simulink model "psbtransfosat"  (Simulink 6.0)
settings: Solver=ode15s  SolverMode=SingleTasking  StartTime=0.0  StopTime=0.5  RelTol=1e-3  AbsTol=1e-2
InitFcn:
  | powericon('psbinitsys',bdroot);
undefined symbols (not defined in the file or in its folder): D1, Delta
libraries: powerlib2 x10, powerlib_extras x1
settings Model: Creator=patrice  LastModifiedBy=batserve  ExtModeTrigMode=oneshot  ExtModeArmWhenConnect=off  ExtModeAutoUpdateStatusClock=off
settings DataIOCC: LimitDataPoints=off  SignalLoggingName=sigsOut
settings OptimizationCC: BlockReduction=off  BooleanDataType=off
settings DebuggingCC: CheckExecutionContextPreStartOutputMsg=on  CheckExecutionContextRuntimeOutputMsg=on  SolverPrmCheckMsg=none  IntegerOverflowMsg=none
settings HardwareCC: TargetUnknown=on
settings RTWCC: TemplateMakefile=grt_unix.tmf

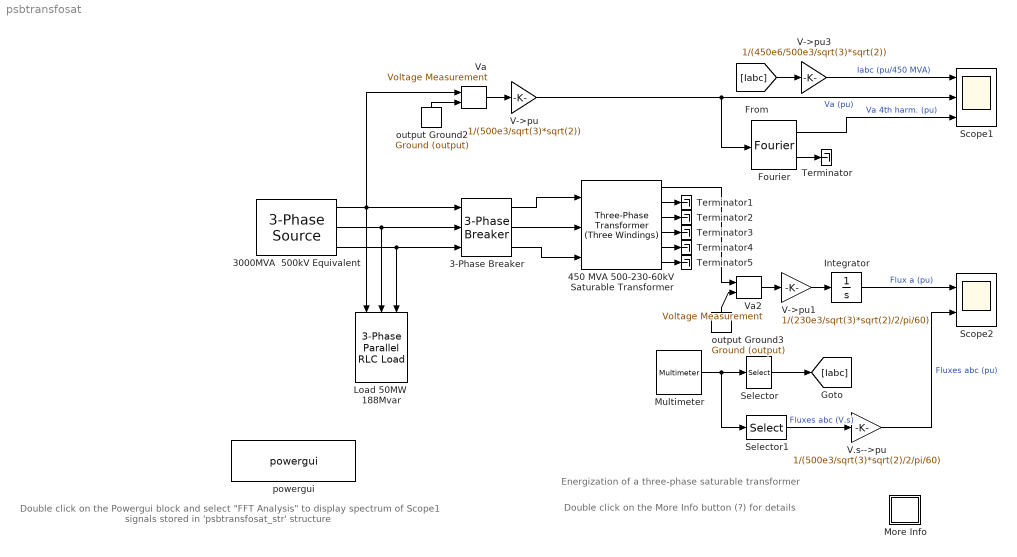
== system psbtransfosat ==
  note: Energization of a three-phase saturable transformer
  note: Double click on the More Info button (?) for details
  note: Double click on the Powergui block and select
      |  "FFT Analysis" to display spectrum of Scope1 signals
      |  stored in 'psbtransfosat_str' structure
  3-Phase Breaker : powerlib2/Elements/3-Phase Breaker  init_states=open  sa=on  sb=on  sc=on  sw_times=[0.05]  Ts=0  comext=off  Ron=0.01  Rp=100e6  Cp=inf  mesure=Breaker currents
  3000MVA  500kV Equivalent : powerlib2/Electrical Sources/3-Phase Source  Tag=PoWeRsYsTeMbLoCk  V=500e3  Phi=0  F=60  InternalConnection=Yg  RLoff=off  R=5.55  L=0.221  Psc=0  Vbase=0  XRratio=0  PSBOutputType=111
  450 MVA 500-230-60kV Saturable Transformer : powerlib2/Elements/Three-Phase Transformer (Three Windings)  Tag=PoWeRsYsTeMbLoCk  confi=ABC as input terminals  nom=[ 450e6 , 60 ]  ydw1=Yg  w1=[ 500e3 0.002 0.08 ]  ydw2=Yg  w2=[ 230e3 0.002 0.08]  ydw3=Delta (D1)  w3=[ 60e3 0.015 0.30]  ynsat=on  rmag=500  lm=500  sat="[0 0; 0.0 1.2; 1.0  1.52]"  hyst=off  matfile='hysteresis'  sif=on  ifl=[0.8 -0.4 0.4]  initialslopes=[+1 +1 +1]  mesure=Fluxes and magnetization currents ( Imag )  PSBOutputType=1111111
  Fourier : powerlib_extras/Measurements/Fourier  f1=60  n=4
  Integrator : Integrator  InitialCondition=0.8  ZeroCross=off
  Load 50MW  188Mvar : powerlib2/Elements/3-Phase Parallel RLC Load  Orientation=down  Vpp=500e3  fn=60  P3=50e6  QL3=0  QC3=188e6
  More Info : Subsystem
      mask Display: disp('?')
  Multimeter : powerlib2/Measurements/Multimeter  Tag=PoWeRsYsTeMmEaSuReMeNt  PhasorSimulation=off  OutputType=Magnitude  sel=[1 2 3 7 8 9]  L=9  Gain=[1 1 1 1 1 1]  yselected={'Ib: 3-Phase Breaker/Breaker A','Ib: 3-Phase Breaker/Breaker B','Ib: 3-Phase Breaker/Breaker C','Flux_A: 450 MVA 500-230-60kV Saturable Transformer','Flux_B: 450 MVA 500-230-60kV Saturable Transformer','Flux_C: 450 MVA 500-230-60kV Saturable Transformer'};  PSBOutputType=1  PSBequivalent=0  AxesSetting=[0,0.1,-100,100]  Display=0  SavedBlockNames={}
  Scope1 : Scope  NumInputPorts=3
      settings: TimeRange=0.5  YMin=-1.5~-1.5~0.05  YMax=3~1.25~0.25  SaveName=psbtransfosat_str  SampleInput=on  SampleTime=1/60/333
  Scope2 : Scope  NumInputPorts=2
      settings: TimeRange=0.5  YMin=-1~-2  YMax=3~3  DataFormat=Structure
  Selector : Selector  Elements=1:3  InputPortWidth=6
  Selector1 : Selector  Elements=4:6  InputPortWidth=6
  Terminator{,1..5} (6 alike) : Terminator
  V->pu : Gain  Gain=1/(500e3/sqrt(3)*sqrt(2))  SaturateOnIntegerOverflow=on
  V->pu1 : Gain  Gain=1/(230e3/sqrt(3)*sqrt(2)/2/pi/60)  SaturateOnIntegerOverflow=on
  V->pu3 : Gain  Gain=1/(450e6/500e3/sqrt(3)*sqrt(2))  SaturateOnIntegerOverflow=on
  V.s-->pu : Gain  Gain=1/(500e3/sqrt(3)*sqrt(2)/2/pi/60)  SaturateOnIntegerOverflow=on
  Va : powerlib2/Measurements/Voltage Measurement  Tag=PoWeRsYsTeMmEaSuReMeNt  PhasorSimulation=off  OutputType=Magnitude  PSBOutputType=0  PSBequivalent=0
  Va2 : powerlib2/Measurements/Voltage Measurement  Tag=PoWeRsYsTeMmEaSuReMeNt  PhasorSimulation=off  OutputType=Magnitude  PSBOutputType=0  PSBequivalent=1
  output Ground2 : powerlib2/Connectors/Ground (output)  Tag=PoWeRsYsTeMbLoCk  Orientation=up  PSBOutputType=1
  output Ground3 : powerlib2/Connectors/Ground (output)  Tag=PoWeRsYsTeMbLoCk  Orientation=up  PSBOutputType=1
  powergui : powerlib2/powergui  Frange=logspace(0,3,50)  Ylog=off  Xlog=off  save=off  variable=ZData  structure=psbtransfosat_str  ZoomFFT=on  StartTime=0.32  cycles=2  DisplayStyle=1  fundamental=60  FreqAxis=on  MaxFrequency=1000  frequencyindice=1  frequencyindicesteady=1  RmsSteady=1  display=off  Ts=0  methode=off  frequency=60  echomessages=off
  wires:
  3000MVA  500kV Equivalent/3 -> Load 50MW  188Mvar/3, 3-Phase Breaker/3
  3000MVA  500kV Equivalent/2 -> Load 50MW  188Mvar/2, 3-Phase Breaker/2
  3000MVA  500kV Equivalent/1 -> Load 50MW  188Mvar/1, Va/1, 3-Phase Breaker/1
  Multimeter/1 -> Selector/1, Selector1/1
  Selector1/1 -> V.s-->pu/1  "Fluxes abc (V.s)"
  output Ground2/1 -> Va/2
  Va/1 -> V->pu/1
  Fourier/2 -> Terminator/1
  Fourier/1 -> Scope1/3  "Va 4th harm. (pu)"
  V->pu/1 -> Fourier/1, Scope1/2  "Va (pu)"
  3-Phase Breaker/1 -> 450 MVA 500-230-60kV Saturable Transformer/1
  3-Phase Breaker/2 -> 450 MVA 500-230-60kV Saturable Transformer/2
  3-Phase Breaker/3 -> 450 MVA 500-230-60kV Saturable Transformer/3
  450 MVA 500-230-60kV Saturable Transformer/1 -> Va2/1
  output Ground3/1 -> Va2/2
  Va2/1 -> V->pu1/1
  V->pu1/1 -> Integrator/1
  Integrator/1 -> Scope2/1  "Flux a (pu)"
  450 MVA 500-230-60kV Saturable Transformer/2 -> Terminator1/1
  450 MVA 500-230-60kV Saturable Transformer/3 -> Terminator2/1
  450 MVA 500-230-60kV Saturable Transformer/4 -> Terminator3/1
  450 MVA 500-230-60kV Saturable Transformer/5 -> Terminator4/1
  450 MVA 500-230-60kV Saturable Transformer/6 -> Terminator5/1
  Selector/1 -> [Iabc]
  [Iabc] -> V->pu3/1
  V->pu3/1 -> Scope1/1  "Iabc (pu/450 MVA)"
  V.s-->pu/1 -> Scope2/2  "Fluxes abc (pu)"

== system psbtransfosat/More Info ==
  note: This demonstration illustrates use of Three-phase, Powergui, and  Multimeter
      | blocks to study  transformer saturation phenomenon
  note: Start the simulation and observe voltage, current and flux waveforms on Scope1 and Scope2.
      |
      | Observe the transformer inrush currents and overvoltage after breaker closing. Because of the 0.8 pu residual flux on phase A and breaker
      | closing at an instant causing maximum flux offset, the flux exceeds 2 pu on phase A. Compare the flux in phase A measured  by the
      | multimeter (yellow trace on 2nd input of Scope2) and the flux obtained by integration of the secondary voltage (first trace of Scope2).
      |
      | Voltage Va  contains a high level of 4th harmonic (displayed on 3rd trace of Scope1) due to the  4th harmonic content of current injected into the
      | network resonating at that particular frequency (max. of 0.23 pu at t = 0.32 s). When  simulation is completed, open the Powergui and select
      | 'FFT Analysis' to display the 0 - 1000 Hz frequency spectrum of signals saved in the 'psbtransfosat_str' structure. The FFT will be performed on
      | a 2-cycle window starting at 0.32 s (instant  of  highest 4th harmonic). Select input labeled 'Va (pu)' and click on Display to obtain the Va voltage spectrum.
      | Notice that  distortion is caused mainly by harmonic orders 2 to 6 (highest content=23% of 4th harmonic as obtained from the Fourier block).
  note: Circuit Description
  note: Demonstration
  note: A three-phase transformer  is energized  on a 500 kV network. The transformer rated 450 MVA, 500 kV/230 kV/60 kV consists of three windings
      | connected in Y/Y/Delta.
      |
      | The power system  is simulated by an equivalent consisting of an  inductive source (short-circuit power of 3000 MVA)  and a parallel RC load.
      | The capacitor reactive power has been selected  in order to produce a  resonance at 240 Hz (4th harmonic).
      |
      | The transformer saturation characteristics is approximated by a single slope Xsat of 0.32 pu, corresponding to  an air core reactance Xac = 0.40 pu
      |  (Xac = Xsat+Xh = 0.32+0.08 = 0.40 pu.) seen from the primary. Three residual fluxes ( -0.8 - 0.4 0.4 pu)  are specified for phases A B and C.
      |
      | The Multimeter and Scope2 blocks are used to monitor extra signals without using  measurement blocks.
      | The six signals obtained at the output of the Multimeter are the three currents in the circuit breaker and the three fluxes inside the
      | core of the saturable transformer. The flux on phase A is also obtained by integrating the  phase A  voltage at the  the unloaded
      | output of winding two. The voltage and flux are converted to p.u. with  gain blocks using proper scaling.
      |
      | A  Simulink masked block named Fourier  measures the 4th harmonic content of the phase A primary voltage
      | This block is available from the Extras/Measurements library.
      |
      | In order to allow further signal processing, signals displayed on Scope1 are sampled at 1/60/333 s (333 samples/ cycle) and stored
      | in a variable named 'psbtransfosat_str'  (structure with time) .
  note: G. Sybille (Hydro-Quebec)
